simulink model "buck_boost"  (R2022a)
settings: Solver=VariableStepAuto  StartTime=0.0  StopTime=0.2  RelTol=1e-3
libraries: spsVoltageMeasurementLib x2, spsSeriesRLCBranchLib x2, spsCurrentMeasurementLib x2, spsIGBTDiodeLib x2, spsParallelRLCBranchLib x2, spsDCVoltageSourceLib x2, spsPWMGeneratorDCDCLib x1, spspowerguiLib x1
settings Model: Creator=jicai  LastModifiedBy=jicai

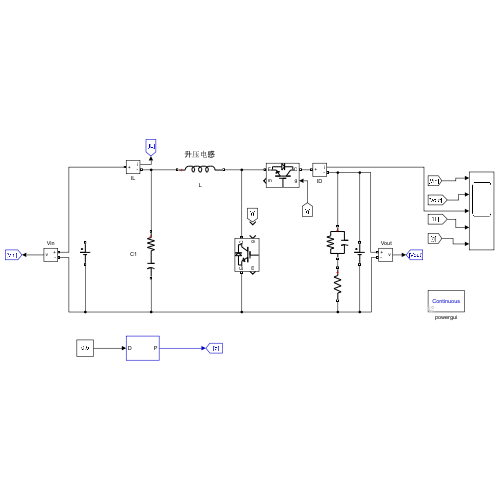
[thumbnail: Simulink's stored preview of the top-level diagram]
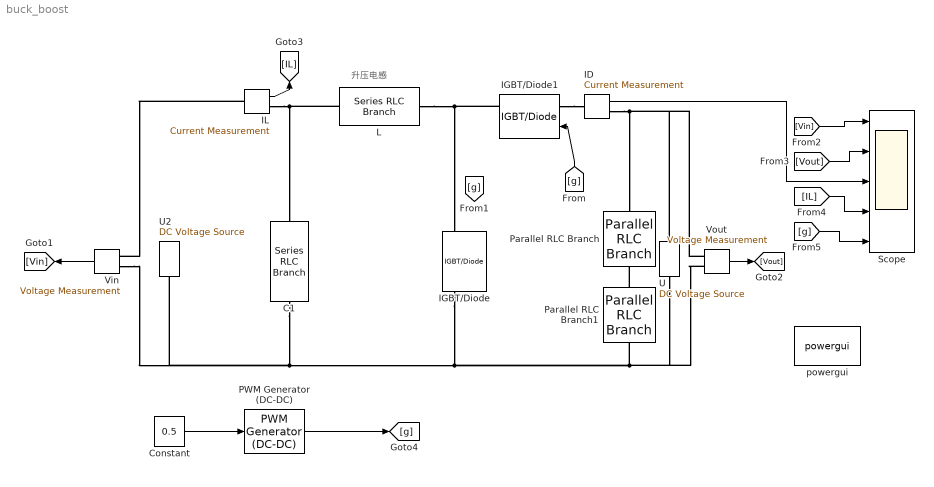
== system buck_boost ==
  note: 升压电感
  " Vout" : spsVoltageMeasurementLib/Voltage Measurement  PhasorSimulation=off  OutputType=Complex  PSBequivalent=0
  C1 : spsSeriesRLCBranchLib/Series RLC Branch  LConnTagsString=__new0  RConnTagsString=__new0  BranchType=RC  Resistance=0.0001  Inductance=5e-3  SetiL0=off  InitialCurrent=0  Capacitance=110e-6  Setx0=off  InitialVoltage=0  Measurements=None
  Constant : Constant  Value=0.5
  ID : spsCurrentMeasurementLib/Current Measurement  PhasorSimulation=off  OutputType=Complex  PSBequivalent=0
  IGBT/Diode : spsIGBTDiodeLib/IGBT//Diode  Ron=1e-3  Rs=1e5  Cs=inf  Measurements=on
  IGBT/Diode1 : spsIGBTDiodeLib/IGBT//Diode  Ron=1e-3  Rs=1e5  Cs=inf  Measurements=on
  IL : spsCurrentMeasurementLib/Current Measurement  PhasorSimulation=off  OutputType=Complex  PSBequivalent=0
  L : spsSeriesRLCBranchLib/Series RLC Branch  LConnTagsString=__new0  RConnTagsString=__new0  BranchType=L  Resistance=1  Inductance=2e-3  SetiL0=off  InitialCurrent=0  Capacitance=1e-6  Setx0=off  InitialVoltage=0  Measurements=None
  PWM Generator (DC-DC) : spsPWMGeneratorDCDCLib/PWM Generator (DC-DC)  Fsw=1e3  Ts=0
  Parallel RLC Branch : spsParallelRLCBranchLib/Parallel RLC Branch  LConnTagsString=a  RConnTagsString=__new0  BranchType=RC  Resistance=10  Inductance=1e-3  SetiL0=off  InitialCurrent=0  Capacitance=100e-6  Setx0=off  InitialVoltage=0  Measurements=None
  Parallel RLC Branch1 : spsParallelRLCBranchLib/Parallel RLC Branch  LConnTagsString=a  RConnTagsString=__new0  BranchType=R  Resistance=0.00001  Inductance=1e-3  SetiL0=off  InitialCurrent=0  Capacitance=100e-6  Setx0=off  InitialVoltage=0  Measurements=None
  Scope : Scope  NumInputPorts=5
  U : spsDCVoltageSourceLib/DC Voltage Source  Amplitude=80  Measurements=None
  U2 : spsDCVoltageSourceLib/DC Voltage Source  Amplitude=100  Measurements=None
  Vin : spsVoltageMeasurementLib/Voltage Measurement  PhasorSimulation=off  OutputType=Complex  PSBequivalent=0
  powergui : spspowerguiLib/powergui  Priority=1  SimulationMode=Continuous  SampleTime=50e-6  frequency=60  Iterations=50  frequencyindice=0  Pbase=100e6  ErrMax=1e-4  UnitsV=kV  UnitsW=MW  buscounter=0  FunctionMessages=off  echomessages=off  EnableUseOfTLC=off  CurrentSourceSwitches=on  DisableSnubberDevices=off  DisableRonSwitches=off  DisableVfSwitches=off  DisplayEquations=off  AutomaticDiscreteSolvers=off  SolverType=Tustin/Backward Euler (TBE)  Interpol=off  ExternalGateDelay=off  methode=off  Ts=10  x0status=blocks  SPID=off  SwTol=0  HookPort=off  NonlinearTolerance=1e-4  nMaxIteration=100  ContinueOnMaxIteration=off  RestoreLinks=warning  ResistiveCurrentMeasurement=off  Frange=[0:2:500]  Ylog=off  Xlog=on  ShowGrid=off  save=off  variable=ZData  structure=0  ZoomFFT=off  StartTime=0.0  cycles=1  DisplayStyle=1  fundamental=60  FreqAxis=off  MaxFrequency=1000  frequencyindicesteady=1  RmsSteady=1  display=off
  wires:
  Constant/1 -> PWM Generator (DC-DC)/1
  " Vout"/1 -> [Vout]
  [Vout] -> Scope/2
  [IL] -> Scope/4
  [Vin] -> Scope/1
  Vin/1 -> [Vin]
  PWM Generator (DC-DC)/1 -> [g]
  [g] -> Scope/5
  IL/1 -> [IL]
  ID/1 -> Scope/3
  [g] -> IGBT/Diode1/1
  connections:
  IL/LConn1 -- Vin/LConn1
  ID/RConn1 -- U/RConn1 -- " Vout"/LConn1 -- Parallel RLC Branch/LConn1
  L/RConn1 -- IGBT/Diode1/RConn1 -- IGBT/Diode/LConn1
  IL/RConn1 -- L/LConn1 -- C1/LConn1
  IGBT/Diode1/LConn1 -- ID/LConn1
  U2/LConn1 -- Vin/LConn2 -- C1/RConn1 -- U/LConn1 -- " Vout"/LConn2 -- Parallel RLC Branch1/RConn1 -- IGBT/Diode/RConn1
  Parallel RLC Branch1/LConn1 -- Parallel RLC Branch/RConn1
